simulink model "BattEv_3motor"  (R2020a)
settings: configuration reference "Reference" (kept outside this file)
undefined symbols (not defined in the file): BattCapInit, BattChargeMax, CapLUTBp, Em, Ns_EV
libraries: autolibdatasheetbattery x1
settings Model: DataDictionary=System_Data_Dictionary.sldd  ModifiedByFormat=The MathWorks, Inc.  PauseTimes=10  OrderedModelArguments=off  Creator=The MathWorks, Inc.  LastModifiedBy=The MathWorks, Inc.
settings ConfigSetRef: SourceName=Reference

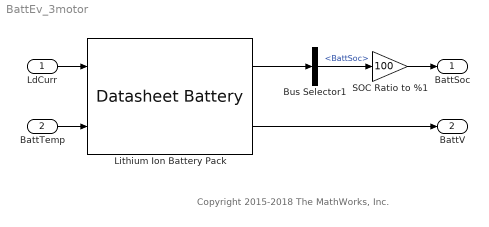
== system BattEv_3motor ==
  note: Copyright 2015-2018 The MathWorks, Inc.
  LdCurr : Inport
  BattTemp : Inport  Port=2
  Bus Selector1 : BusSelector  OutputSignals=BattSoc
  Lithium Ion Battery Pack : autolibdatasheetbattery/Datasheet Battery  CapacityCtrl=Parameter  OutputVlt=Filtered  BattChargeMax=BattChargeMax  Em=Em  CapLUTBp=CapLUTBp  RInt=RInt  BattTempBp=BattTempBp  CapSOCBp=CapSOCBp  Ns=Ns_EV  Np=Np_EV  BattCapInit=BattCapInit_EV  Tc=Tc_Batt  Vinit=Ns_EV*interp1(CapLUTBp, Em, BattCapInit/BattChargeMax)  RefBlkName='autolibdatasheetbattery/Datasheet Battery'
      settings: SourceProductBaseCode=PW
  SOC Ratio to %1 : Gain  Gain=100
  BattSoc : Outport  VectorParamsAs1DForOutWhenUnconnected=off
  BattV : Outport  Port=2  VectorParamsAs1DForOutWhenUnconnected=off
  wires:
  BattTemp/1 -> Lithium Ion Battery Pack/2
  Lithium Ion Battery Pack/1 -> Bus Selector1/1
  Bus Selector1/1 -> SOC Ratio to %1/1  "<BattSoc>"
  SOC Ratio to %1/1 -> BattSoc/1
  Lithium Ion Battery Pack/2 -> BattV/1
  LdCurr/1 -> Lithium Ion Battery Pack/1
